simulink model "lab4_1"  (R2018a)
settings: Solver=ode45  StartTime=0.0  StopTime=15  MaxStep=0.001  RelTol=1e-3
settings Model: Creator=Koala  LastModifiedBy=Koala

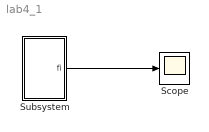
== system lab4_1 ==
  Scope : Scope
  Subsystem : Subsystem  mask{m=2, k=2, g=9.81, l=1, fi0=90}
  wires:
  Subsystem/1(fi) -> Scope/1

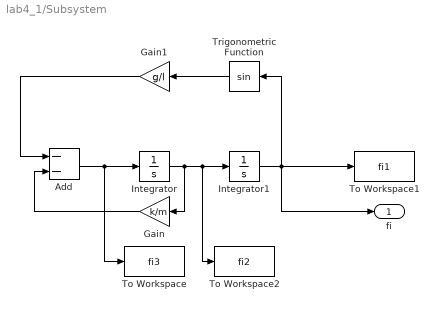
== system lab4_1/Subsystem ==
  Add : Sum  Inputs=--
  Gain : Gain  Gain=k/m
  Gain1 : Gain  Gain=g/l
  Integrator : Integrator
  Integrator1 : Integrator  InitialCondition=fi0*pi/180
  To Workspace : ToWorkspace  VariableName=fi3  SampleTime=-1
  To Workspace1 : ToWorkspace  VariableName=fi1  SampleTime=-1
  To Workspace2 : ToWorkspace  VariableName=fi2  SampleTime=-1
  Trigonometric Function : Trigonometry
  fi : Outport
  wires:
  Gain/1 -> Add/2
  Integrator1/1 -> fi/1, To Workspace1/1, Trigonometric Function/1
  Add/1 -> To Workspace/1, Integrator/1
  Integrator/1 -> Gain/1, To Workspace2/1, Integrator1/1
  Trigonometric Function/1 -> Gain1/1
  Gain1/1 -> Add/1
